simulink model "flexible_joint_v4_rl_Slave_Action_2025"  (R2023b)
settings: Solver=FixedStepAuto  StartTime=0.0  StopTime=40  FixedStep=0.001  RelTol=1e-3
undefined symbols (not defined in the file): DiscIntNeverNeededParam, epsilon, Kmin, LIMIT_SATURATE, NOISE_ADD
libraries: simulink x6, rllib x1
settings Model: Creator=GreenTeam  LastModifiedBy=GreenTeam
settings DataIOCC: InspectSignalLogs=on

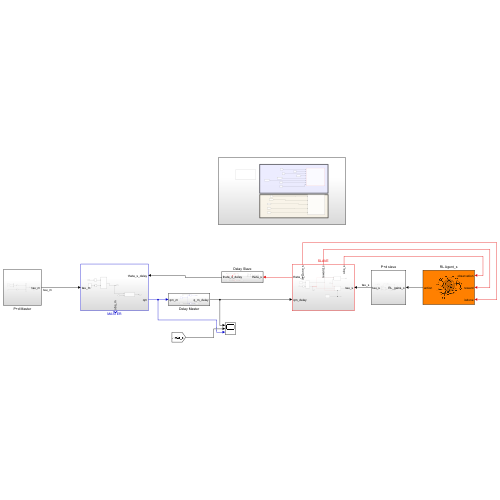
[thumbnail: Simulink's stored preview of the top-level diagram]
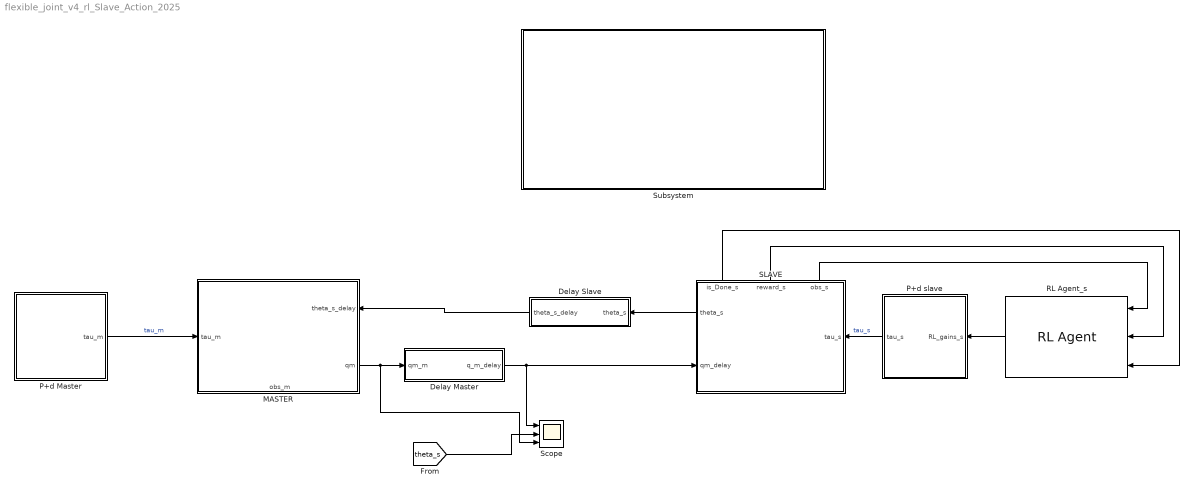
== system flexible_joint_v4_rl_Slave_Action_2025 ==
  Delay Master : Subsystem
  Delay Slave : Subsystem
  MASTER : Subsystem
      settings: PortSchema="{\"entries\":[{\"content\":{\"sides\":[{\"content\":{\"connectorIds\":[\"In1\"]},\"type\":\"ConnectorPlacement.EquallySpacedRectSide\",\"uuid\":\"b129d543-5df5-48a3-934f-a2bf4f7acba4\"},{\"content\":{\"connectorIds\":[\"In2\",\"Out1\"],\"side\":\"RIGHT\"},\"type\":\"ConnectorPlacement.EquallySpacedRectSide\",\"uuid\":\"06efd871-fa3f-497a-8ca9-8980933123ca\"},{\"content\":{\"side\":\"TOP\"},\"type\":\"ConnectorPlacement.EquallySpacedRectSide\",\"uuid\":\"af305e1d-4707-4128-8291-282686c4f98c\"},{\"content\":{\"connectorIds\":[\"Out2\"],\"side\":\"BOTTOM\"},\"type\":\"ConnectorPlacement.EquallySpacedRectSide\",\"uuid\":\"179bfa12-bc3e-4c80-81e3-e51d757695b6\"}]},\"type\":\"ConnectorPlacement.EquallySpacedConnector\",\"uuid\":\"58b08623-3413-4316-b8cd-a4fc96e4577b\"}],\"packageUris\":[\"http://schema.mathworks.com/mf0/Connector/R2020b\"],\"version\":\"1.0\"}"
  P+d Master : Subsystem
  P+d slave : Subsystem
  RL Agent_s : rllib/RL Agent  Agent=agent_s  ExternalActionAsInput=off  ProvideLastAction=off  ProvideCumRwd=off  TreatAsDirectFeedthrough=on  UseStrictObservationDataTypes=off
  SLAVE : Subsystem
      settings: PortSchema="{\"entries\":[{\"content\":{\"sides\":[{\"content\":{\"connectorIds\":[\"In1\"]},\"type\":\"ConnectorPlacement.EquallySpacedRectSide\",\"uuid\":\"b129d543-5df5-48a3-934f-a2bf4f7acba4\"},{\"content\":{\"connectorIds\":[\"Out1\",\"In2\"],\"side\":\"RIGHT\"},\"type\":\"ConnectorPlacement.EquallySpacedRectSide\",\"uuid\":\"06efd871-fa3f-497a-8ca9-8980933123ca\"},{\"content\":{\"connectorIds\":[\"Out2\",\"Out3\",\"Out4\"],\"side\":\"TOP\"},\"type\":\"ConnectorPlacement.EquallySpacedRectSide\",\"uuid\":\"af305e1d-4707-4128-8291-282686c4f98c\"},{\"content\":{\"side\":\"BOTTOM\"},\"type\":\"ConnectorPlacement.EquallySpacedRectSide\",\"uuid\":\"f24c9865-98ea-4837-b1c7-54c0879e04e0\"}]},\"type\":\"ConnectorPlacement.EquallySpacedConnector\",\"uuid\":\"58b08623-3413-4316-b8cd-a4fc96e4577b\"}],\"packageUris\":[\"http://schema.mathworks.com/mf0/Connector/R2020b\"],\"version\":\"1.0\"}"
  Scope : Scope  NumInputPorts=3
  Subsystem : Subsystem
  wires:
  P+d Master/1(tau_m) -> MASTER/1(tau_m)  "tau_m"
  MASTER/1(qm) -> Scope/3, Delay Master/1(qm_m)
  Delay Slave/1(theta_s_delay) -> MASTER/2(theta_s_delay)
  Delay Master/1(q_m_delay) -> Scope/1, SLAVE/2(qm_delay)
  SLAVE/1(theta_s) -> Delay Slave/1(theta_s)
  SLAVE/2(obs_s) -> RL Agent_s/1
  SLAVE/3(reward_s) -> RL Agent_s/2
  SLAVE/4(is_Done_s) -> RL Agent_s/3
  RL Agent_s/1 -> P+d slave/1(RL_gains_s)
  P+d slave/1(tau_s) -> SLAVE/1(tau_s)  "tau_s"
  [theta_s] -> Scope/2

== system flexible_joint_v4_rl_Slave_Action_2025/Delay Master ==
  qm_m : Inport
  Variable Time Delay1 : VariableTransportDelay  MaximumDelay=10  MaximumPoints=499712
  Variable Time Delay5 : VariableTransportDelay  MaximumDelay=10  MaximumPoints=499712
  delay_m : Subsystem
  q_m_delay : Outport
  tag scope: dqm_delay=global
  wires:
  Variable Time Delay5/1 -> q_m_delay/1
  qm_m/1 -> Variable Time Delay5/1
  [dqm] -> Variable Time Delay1/1
  Variable Time Delay1/1 -> [dqm_delay]
  delay_m/1(d) -> Variable Time Delay1/2, Variable Time Delay5/2

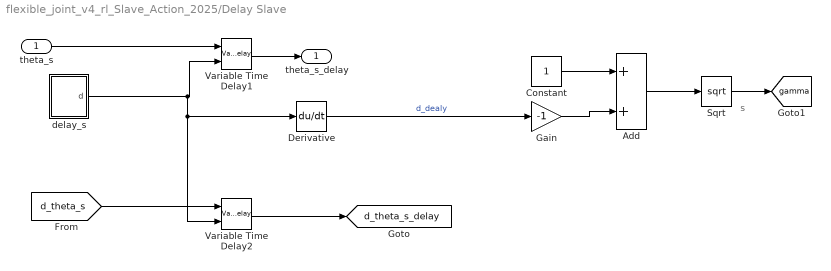
== system flexible_joint_v4_rl_Slave_Action_2025/Delay Slave ==
  note: s
  theta_s : Inport
  Add : Sum
  Constant : Constant
  Derivative : Derivative
  Gain : Gain  Gain=-1
  Sqrt : Sqrt
  Variable Time Delay1 : VariableTransportDelay  MaximumDelay=10  MaximumPoints=499712
  Variable Time Delay2 : VariableTransportDelay  MaximumDelay=10  MaximumPoints=499712
  delay_s : Subsystem
  theta_s_delay : Outport
  tag scope: d_theta_s_delay=global, gamma=global
  wires:
  Variable Time Delay1/1 -> theta_s_delay/1
  theta_s/1 -> Variable Time Delay1/1
  delay_s/1(d) -> Derivative/1, Variable Time Delay2/2, Variable Time Delay1/2
  [d_theta_s] -> Variable Time Delay2/1
  Variable Time Delay2/1 -> [d_theta_s_delay]
  Derivative/1 -> Gain/1  "d_dealy"
  Constant/1 -> Add/1
  Gain/1 -> Add/2
  Add/1 -> Sqrt/1
  Sqrt/1 -> [gamma]

== system flexible_joint_v4_rl_Slave_Action_2025/MASTER ==
  tau_m : Inport
  theta_s_delay : Inport  Port=2
  Master : Subsystem
  Observation : Subsystem
  Saturation1 : Saturate  UpperLimit=LIMIT_SATURATE  LowerLimit=-1*LIMIT_SATURATE
  Saturation2 : Saturate  UpperLimit=LIMIT_SATURATE  LowerLimit=-1*LIMIT_SATURATE
  tauh : Subsystem
  qm : Outport
  obs_m : Outport  Port=2
  wires:
  tauh/1(out) -> Saturation2/1
  tau_m/1 -> Saturation1/1
  Master/1(qm) -> Observation/1(q_m), qm/1
  theta_s_delay/1 -> Observation/2(theta_s_delay)
  Observation/1(observeation) -> obs_m/1
  Saturation2/1 -> Master/2(tau_h)
  Saturation1/1 -> Master/1(tau_m)

== system flexible_joint_v4_rl_Slave_Action_2025/P+d Master ==
  Bm : Gain  Gain=5
  Gain : Gain
  Km : Gain  Gain=5
  Mux2 : Mux  Inputs=2
  Subtract1 : Sum
  tau_m : Outport
  tag scope: tau_m=global
  wires:
  Subtract1/1 -> Gain/1
  Gain/1 -> [tau_m], tau_m/1
  [error_m] -> Km/1
  [dqm_1] -> Mux2/1
  [dqm_2] -> Mux2/2
  Mux2/1 -> Bm/1
  Bm/1 -> Subtract1/1
  Km/1 -> Subtract1/2

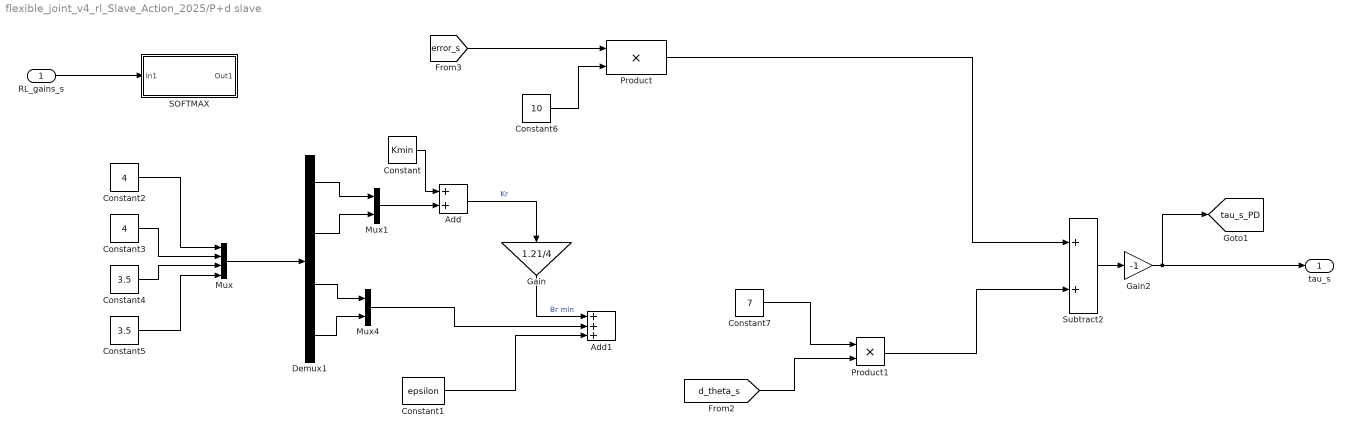
== system flexible_joint_v4_rl_Slave_Action_2025/P+d slave ==
  RL_gains_s : Inport
  Add : Sum
  Add1 : Sum  Inputs=+++
  Constant : Constant  Value=Kmin
  Constant1 : Constant  Value=epsilon
  Constant2 : Constant  Value=4
  Constant3 : Constant  Value=4
  Constant4 : Constant  Value=3.5
  Constant5 : Constant  Value=3.5
  Constant6 : Constant  Value=10
  Constant7 : Constant  Value=7
  Demux1 : Demux
  Gain : Gain  Gain=1.21/4
  Gain2 : Gain  Gain=-1
  Mux : Mux
  Mux1 : Mux  Inputs=2
  Mux4 : Mux  Inputs=2
  Product : Product
  Product1 : Product
  SOFTMAX : Subsystem
  Subtract2 : Sum
  tau_s : Outport
  tag scope: tau_s_PD=global
  wires:
  Subtract2/1 -> Gain2/1
  Gain2/1 -> tau_s/1, [tau_s_PD]
  [error_s] -> Product/1
  Demux1/1 -> Mux1/1
  Demux1/2 -> Mux1/2
  Demux1/3 -> Mux4/1
  Demux1/4 -> Mux4/2
  RL_gains_s/1 -> SOFTMAX/1(In1)
  Mux1/1 -> Add/2
  Constant/1 -> Add/1
  Add/1 -> Gain/1  "Kr"
  Gain/1 -> Add1/1  "Br min"
  Mux4/1 -> Add1/2
  Constant1/1 -> Add1/3
  Product/1 -> Subtract2/1
  Product1/1 -> Subtract2/2
  [d_theta_s] -> Product1/2
  Mux/1 -> Demux1/1
  Constant2/1 -> Mux/1
  Constant5/1 -> Mux/4
  Constant3/1 -> Mux/2
  Constant4/1 -> Mux/3
  Constant6/1 -> Product/2
  Constant7/1 -> Product1/1

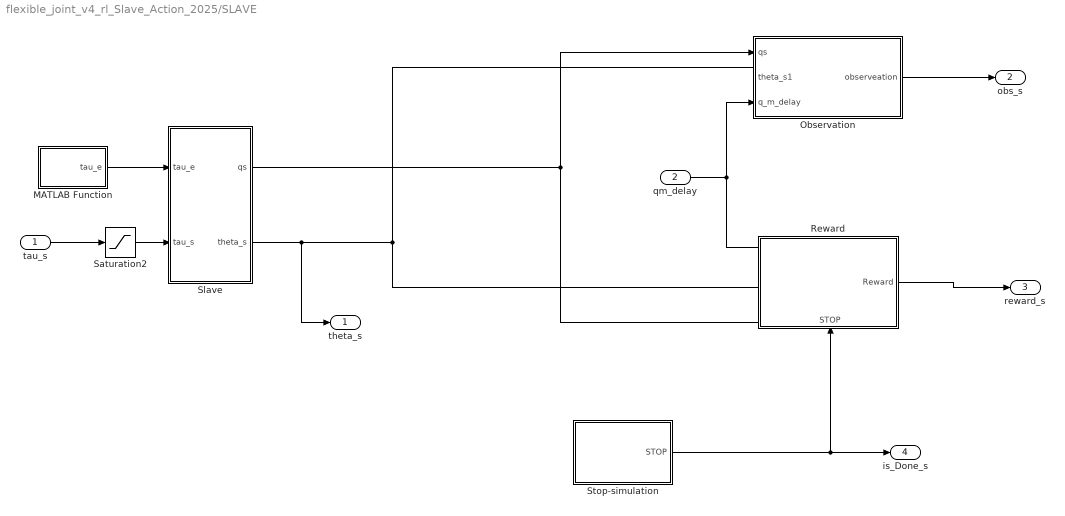
== system flexible_joint_v4_rl_Slave_Action_2025/SLAVE ==
  tau_s : Inport
  qm_delay : Inport  Port=2
  MATLAB Function : MATLAB Function  TreatAsAtomicUnit=on
  Observation : Subsystem
  Reward : Subsystem
      settings: PortSchema="{\"entries\":[{\"content\":{\"sides\":[{\"content\":{},\"type\":\"ConnectorPlacement.EquallySpacedRectSide\",\"uuid\":\"9a737741-b920-4653-b681-b634863af948\"},{\"content\":{\"connectorIds\":[\"Out1\"],\"side\":\"RIGHT\"},\"type\":\"ConnectorPlacement.EquallySpacedRectSide\",\"uuid\":\"0a2b46ef-cff1-47c3-8c56-381f72c27921\"},{\"content\":{\"side\":\"TOP\"},\"type\":\"ConnectorPlacement.EquallySpacedRectSide\",\"uuid\":\"0d3246b3-4748-4708-b0d4-097592cf6e81\"},{\"content\":{\"connectorIds\":[\"In1\"],\"side\":\"BOTTOM\"},\"type\":\"ConnectorPlacement.EquallySpacedRectSide\",\"uuid\":\"566fc9c6-ad4c-440d-8570-c1b5e2d37a92\"}]},\"type\":\"ConnectorPlacement.EquallySpacedConnector\",\"uuid\":\"b2a81796-0154-474c-b467-1f1d418e5717\"}],\"packageUris\":[\"http://schema.mathworks.com/mf0/Connector/R2020b\"],\"version\":\"1.0\"}"
  Saturation2 : Saturate  UpperLimit=LIMIT_SATURATE  LowerLimit=-1*LIMIT_SATURATE
  Slave : Subsystem
  Stop-simulation : Subsystem
  theta_s : Outport
  obs_s : Outport  Port=2
  reward_s : Outport  Port=3
  is_Done_s : Outport  Port=4
  wires:
  MATLAB Function/1(tau_e) -> Slave/1(tau_e)
  tau_s/1 -> Saturation2/1
  Slave/1(qs) -> Observation/1(qs)
  Reward/1(Reward) -> reward_s/1
  Slave/2(theta_s) -> theta_s/1
  qm_delay/1 -> Observation/3(q_m_delay)
  Observation/1(observeation) -> obs_s/1
  Stop-simulation/1(STOP) -> is_Done_s/1, Reward/1(STOP)
  Saturation2/1 -> Slave/2(tau_s)

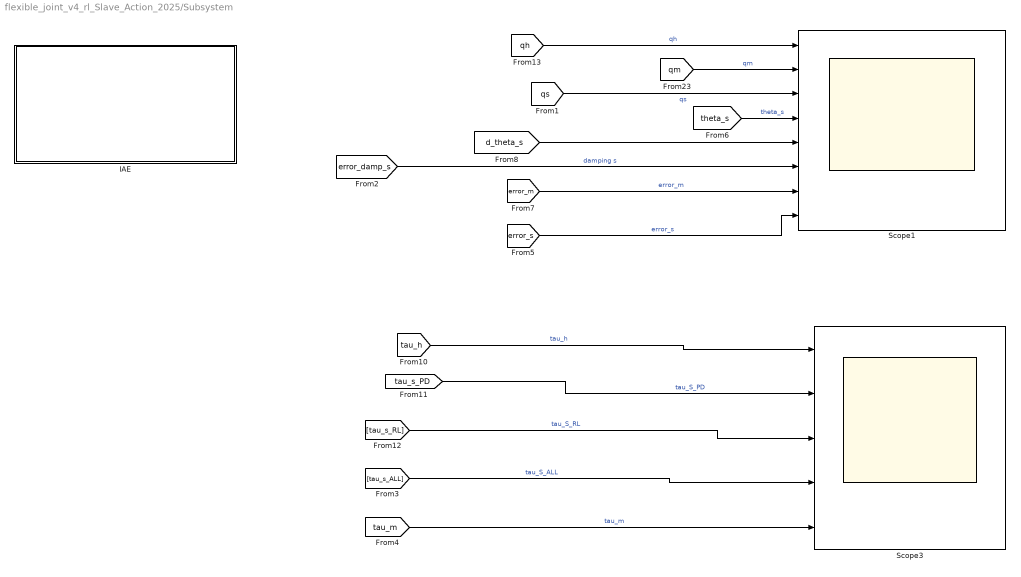
== system flexible_joint_v4_rl_Slave_Action_2025/Subsystem ==
  IAE : Subsystem
  Scope1 : Scope  NumInputPorts=8
  Scope3 : Scope  NumInputPorts=5
  wires:
  [qh] -> Scope1/1  "qh"
  [qm] -> Scope1/2  "qm"
  [error_damp_s] -> Scope1/6  "damping s"
  [error_m] -> Scope1/7  "error_m"
  [error_s] -> Scope1/8  "error_s"
  [qs] -> Scope1/3  "qs"
  [theta_s] -> Scope1/4  "theta_s"
  [d_theta_s] -> Scope1/5
  [tau_s_PD] -> Scope3/2  "tau_S_PD"
  [tau_h] -> Scope3/1  "tau_h"
  [tau_s_RL] -> Scope3/3  "tau_S_RL"
  [tau_s_ALL] -> Scope3/4  "tau_S_ALL"
  [tau_m] -> Scope3/5  "tau_m"

== system flexible_joint_v4_rl_Slave_Action_2025/Delay Master/delay_m ==
  Clock : Clock
  Gain_delay_m : Gain  Gain=0.86907
  MATLAB Function : MATLAB Function  TreatAsAtomicUnit=on
  Scope : Scope
  d : Outport
  wires:
  MATLAB Function/1(y) -> Scope/1, Gain_delay_m/1
  Clock/1 -> MATLAB Function/1(t)
  Gain_delay_m/1 -> d/1

== system flexible_joint_v4_rl_Slave_Action_2025/Delay Slave/delay_s ==
  Clock : Clock
  Gain_delay_s : Gain  Gain=0.73854
  MATLAB Function : MATLAB Function  TreatAsAtomicUnit=on
  d : Outport
  wires:
  Clock/1 -> MATLAB Function/1(t)
  MATLAB Function/1(y) -> Gain_delay_s/1
  Gain_delay_s/1 -> d/1

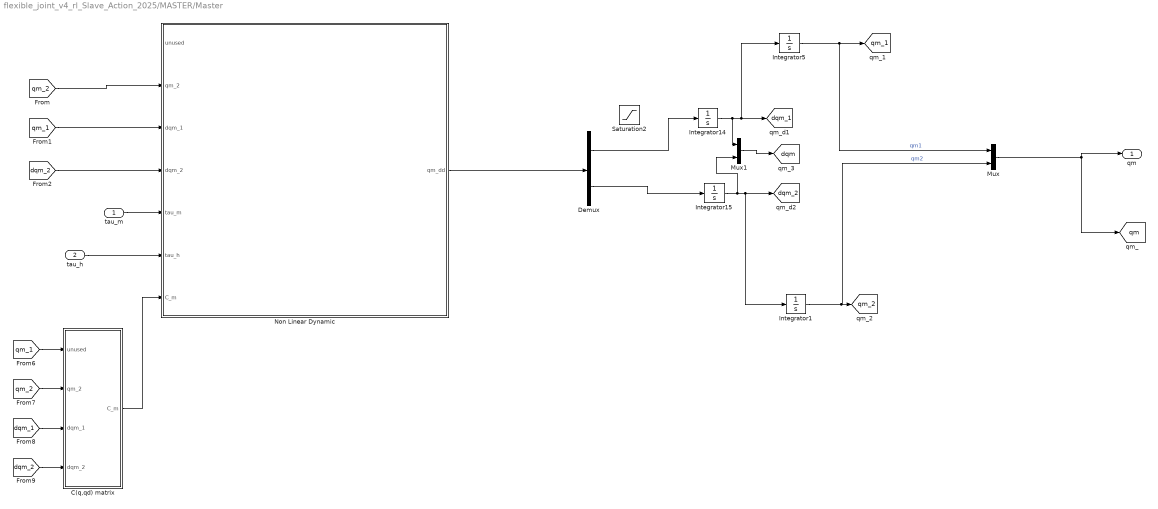
== system flexible_joint_v4_rl_Slave_Action_2025/MASTER/Master ==
  tau_m : Inport
  tau_h : Inport  Port=2
  C(q,qd) matrix : MATLAB Function  TreatAsAtomicUnit=on
  Demux : Demux  Outputs=2
  Integrator1 : Integrator  InitialCondition=1/5
  Integrator14 : Integrator
  Integrator15 : Integrator
  Integrator5 : Integrator  InitialCondition=-1/5
  Mux : Mux  Inputs=2
  Mux1 : Mux  Inputs=2
  Non Linear Dynamic : MATLAB Function  TreatAsAtomicUnit=on
  Saturation2 : Saturate  UpperLimit=1000000  LowerLimit=1000000*-1
  qm : Outport  VectorParamsAs1DForOutWhenUnconnected=off
  tag scope: dqm=global, dqm_1=global, dqm_2=global, qm=global, qm_1=global, qm_2=global
  wires:
  Integrator5/1 -> Mux/1, [qm_1]  "qm1"
  Demux/1 -> Integrator14/1
  Non Linear Dynamic/1(qm_dd) -> Demux/1
  Integrator1/1 -> Mux/2, [qm_2]  "qm2"
  tau_m/1 -> Non Linear Dynamic/5(tau_m)
  Integrator14/1 -> Mux1/1, Integrator5/1, [dqm_1]
  Integrator15/1 -> Mux1/2, Integrator1/1, [dqm_2]
  C(q,qd) matrix/1(C_m) -> Non Linear Dynamic/7(C_m)
  [qm_2] -> Non Linear Dynamic/2(qm_2)
  [dqm_2] -> Non Linear Dynamic/4(dqm_2)
  [qm_1] -> Non Linear Dynamic/3(dqm_1)
  [dqm_1] -> C(q,qd) matrix/3(dqm_1)
  [qm_1] -> C(q,qd) matrix/1(unused)
  [dqm_2] -> C(q,qd) matrix/4(dqm_2)
  [qm_2] -> C(q,qd) matrix/2(qm_2)
  tau_h/1 -> Non Linear Dynamic/6(tau_h)
  Mux1/1 -> [dqm]
  Demux/2 -> Integrator15/1
  Mux/1 -> qm/1, [qm]

== system flexible_joint_v4_rl_Slave_Action_2025/MASTER/Observation ==
  q_m : Inport
  theta_s_delay : Inport  Port=2
  Subtract : Sum  Inputs=+-
  observeation : Outport
  tag scope: error_m=global
  wires:
  q_m/1 -> Subtract/1
  theta_s_delay/1 -> Subtract/2
  Subtract/1 -> [error_m]

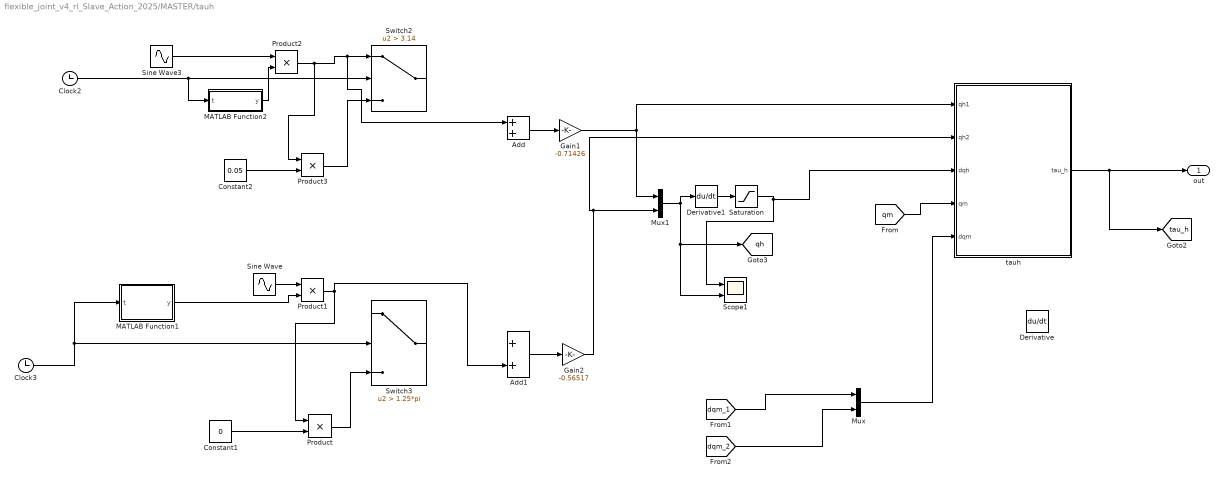
== system flexible_joint_v4_rl_Slave_Action_2025/MASTER/tauh ==
  Add : Sum
  Add1 : Sum
  Clock2 : Clock
  Clock3 : Clock
  Constant1 : Constant  Value=0
  Constant2 : Constant  Value=0.05
  Derivative : Derivative
  Derivative1 : Derivative
  Gain1 : Gain  Gain=-0.71426
  Gain2 : Gain  Gain=-0.56517
  MATLAB Function1 : MATLAB Function  TreatAsAtomicUnit=on
  MATLAB Function2 : MATLAB Function  TreatAsAtomicUnit=on
  Mux : Mux  Inputs=2
  Mux1 : Mux  Inputs=2
  Product{,1..3} (4 alike) : Product
  Saturation : Saturate  UpperLimit=1  LowerLimit=-1
  Scope1 : Scope  NumInputPorts=2
  Sine Wave : Sin  Amplitude=2.5  Frequency=1.6  Phase=0.05  SampleTime=0
  Sine Wave3 : Sin  Amplitude=3  SampleTime=0
  Switch2 : Switch  Criteria=u2 > Threshold  Threshold=3.14  SaturateOnIntegerOverflow=off  InputSameDT=off
  Switch3 : Switch  Criteria=u2 > Threshold  Threshold=1.25*pi  SaturateOnIntegerOverflow=off  InputSameDT=off
  tauh : MATLAB Function  TreatAsAtomicUnit=on
  out : Outport
  tag scope: qh=global, tau_h=global
  wires:
  tauh/1(tau_h) -> [tau_h], out/1
  [dqm_1] -> Mux/1
  [dqm_2] -> Mux/2
  Mux/1 -> tauh/5(dqm)
  [qm] -> tauh/4(qm)
  Mux1/1 -> Scope1/2, [qh], Derivative1/1
  Clock3/1 -> Switch3/2, MATLAB Function1/1(t)
  Clock2/1 -> MATLAB Function2/1(t), Switch2/2
  Add/1 -> Gain1/1
  MATLAB Function1/1(y) -> Product1/2
  Sine Wave/1 -> Product1/1
  Add1/1 -> Gain2/1
  Gain1/1 -> tauh/1(qh1), Mux1/1
  Sine Wave3/1 -> Product2/1
  MATLAB Function2/1(y) -> Product2/2
  Product2/1 -> Product3/1, Add/1, Switch2/1
  Product1/1 -> Product/1, Add1/2
  Derivative1/1 -> Saturation/1
  Saturation/1 -> Scope1/1, tauh/3(dqh)
  Constant1/1 -> Product/2
  Product/1 -> Switch3/3
  Constant2/1 -> Product3/2
  Product3/1 -> Switch2/3
  Gain2/1 -> tauh/2(qh2), Mux1/2

== system flexible_joint_v4_rl_Slave_Action_2025/P+d slave/SOFTMAX ==
  In1 : Inport
  Add : Sum
  Constant : Constant
  Exp : Math
  Log : Math  Operator=log
  Out1 : Outport
  wires:
  Log/1 -> Out1/1
  Constant/1 -> Add/1
  Exp/1 -> Add/2
  In1/1 -> Exp/1
  Add/1 -> Log/1

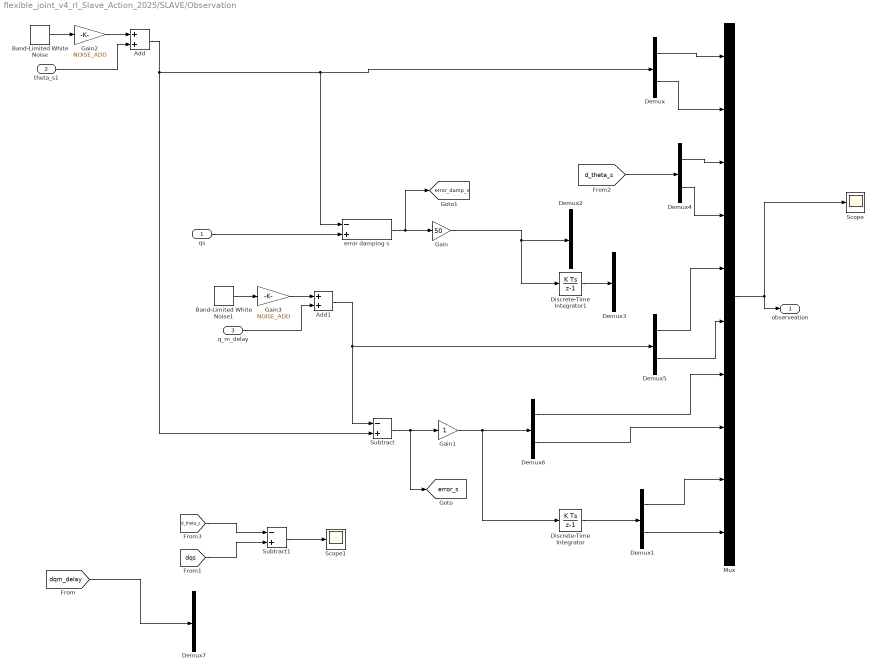
== system flexible_joint_v4_rl_Slave_Action_2025/SLAVE/Observation ==
  qs : Inport
  theta_s1 : Inport  Port=2
  q_m_delay : Inport  Port=3
  Add : Sum
  Add1 : Sum
  Band-Limited White Noise : simulink/Sources/Band-Limited White Noise  Cov=[0.005]  Ts=0.01  seed=[23341]
  Band-Limited White Noise1 : simulink/Sources/Band-Limited White Noise  Cov=[0.005]  Ts=0.01  seed=[23341]
  Demux{,1..7} (8 alike) : Demux  Outputs=2
  Discrete-Time Integrator : DiscreteIntegrator  SampleTime=-1  ICPrevOutput=DiscIntNeverNeededParam  ICPrevScaledInput=DiscIntNeverNeededParam
  Discrete-Time Integrator1 : DiscreteIntegrator  SampleTime=-1  ICPrevOutput=DiscIntNeverNeededParam  ICPrevScaledInput=DiscIntNeverNeededParam
  Gain : Gain  Gain=50
  Gain1 : Gain
  Gain2 : Gain  Gain=NOISE_ADD
  Gain3 : Gain  Gain=NOISE_ADD
  Mux : Mux  Inputs=10
  Scope : Scope
  Scope1 : Scope
  Subtract : Sum  Inputs=-+
  Subtract1 : Sum  Inputs=-+
  error damping s : Sum  Inputs=-+
  observeation : Outport
  tag scope: error_damp_s=global, error_s=global
  wires:
  Discrete-Time Integrator/1 -> Demux1/1
  Mux/1 -> Scope/1, observeation/1
  Add/1 -> Subtract/2, error damping s/1, Demux/1
  [d_theta_s] -> Demux4/1
  qs/1 -> error damping s/2
  Discrete-Time Integrator1/1 -> Demux3/1
  error damping s/1 -> [error_damp_s], Gain/1
  [dqm_delay] -> Demux7/1
  Subtract/1 -> [error_s], Gain1/1
  Gain/1 -> Discrete-Time Integrator1/1, Demux2/1
  Demux/1 -> Mux/1
  Demux/2 -> Mux/2
  Demux4/1 -> Mux/3
  Demux4/2 -> Mux/4
  Demux5/1 -> Mux/5
  Demux5/2 -> Mux/6
  Gain1/1 -> Discrete-Time Integrator/1, Demux6/1
  [dqs] -> Subtract1/2
  [d_theta_s] -> Subtract1/1
  Subtract1/1 -> Scope1/1
  Demux6/1 -> Mux/7
  Demux6/2 -> Mux/8
  Demux1/1 -> Mux/9
  Demux1/2 -> Mux/10
  Band-Limited White Noise/1 -> Gain2/1
  Gain2/1 -> Add/1
  theta_s1/1 -> Add/2
  Band-Limited White Noise1/1 -> Gain3/1
  q_m_delay/1 -> Add1/2
  Gain3/1 -> Add1/1
  Add1/1 -> Subtract/1, Demux5/1

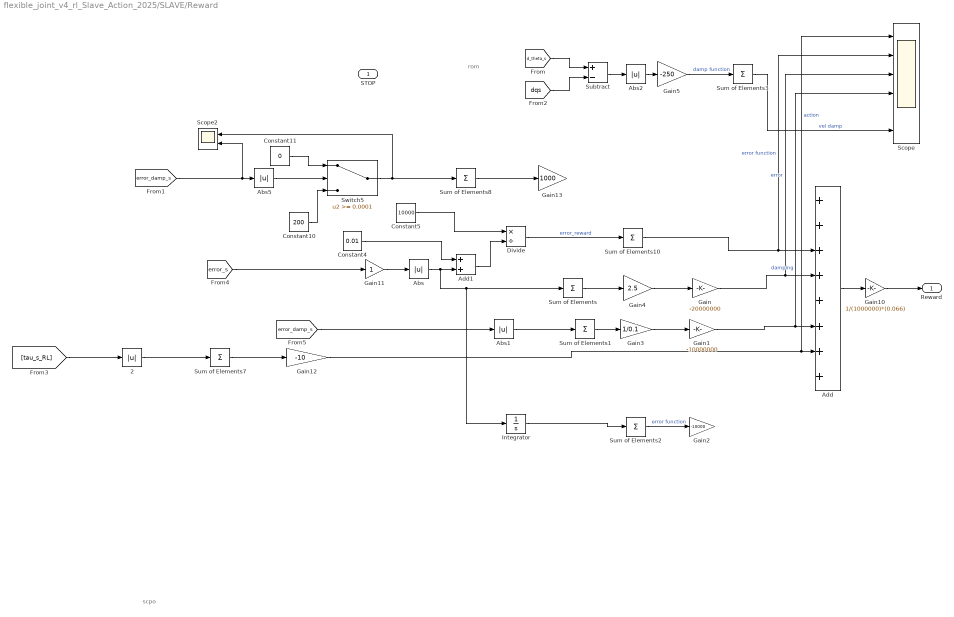
== system flexible_joint_v4_rl_Slave_Action_2025/SLAVE/Reward ==
  note: rom
  note: scpo
  STOP : Inport
  " 2" : Abs  SaturateOnIntegerOverflow=off
  Abs{,1..2,5} (4 alike) : Abs  SaturateOnIntegerOverflow=off
  Add : Sum  Inputs=++++++++
  Add1 : Sum
  Constant10 : Constant  Value=200
  Constant11 : Constant  Value=0
  Constant4 : Constant  Value=0.01
  Constant5 : Constant  Value=10000
  Divide : Product  Inputs=*/
  Gain : Gain  Gain=-20000000
  Gain1 : Gain  Gain=-10000000
  Gain10 : Gain  Gain=1/(1000000)*(0.066)
  Gain11 : Gain
  Gain12 : Gain  Gain=-10
  Gain13 : Gain  Gain=1000
  Gain2 : Gain  Gain=-10000
  Gain3 : Gain  Gain=1/0.1
  Gain4 : Gain  Gain=2.5
  Gain5 : Gain  Gain=-250
  Integrator : Integrator
  Scope : Scope  NumInputPorts=6
  Scope2 : Scope  NumInputPorts=2
  Subtract : Sum  Inputs=+-
  Sum of Elements{,1..3,7..8,10} (7 alike) : Sum  Inputs=+
  Switch5 : Switch  Threshold=0.0001  SaturateOnIntegerOverflow=off  InputSameDT=off
  Reward : Outport
  wires:
  Sum of Elements/1 -> Gain4/1
  Gain4/1 -> Gain/1
  Sum of Elements1/1 -> Gain3/1
  Gain3/1 -> Gain1/1
  Abs1/1 -> Sum of Elements1/1
  [error_damp_s] -> Abs1/1
  Add/1 -> Gain10/1
  Gain10/1 -> Reward/1
  Abs/1 -> Integrator/1, Sum of Elements/1, Add1/2
  Constant4/1 -> Add1/1
  Add1/1 -> Divide/2
  Constant5/1 -> Divide/1
  Gain11/1 -> Abs/1
  [error_s] -> Gain11/1
  [tau_s_RL] -> " 2"/1
  Sum of Elements7/1 -> Gain12/1
  Gain12/1 -> Scope/1, Add/7  "action"
  [error_damp_s] -> Abs5/1, Scope2/2
  Constant10/1 -> Switch5/3
  Constant11/1 -> Switch5/1
  Switch5/1 -> Sum of Elements8/1, Scope2/1
  Sum of Elements8/1 -> Gain13/1
  Divide/1 -> Sum of Elements10/1  "error_reward"
  Abs5/1 -> Switch5/2
  " 2"/1 -> Sum of Elements7/1
  Gain1/1 -> Scope/4, Add/6  "damping"
  Sum of Elements10/1 -> Scope/2, Add/3  "error function"
  Gain/1 -> Scope/3, Add/4  "error"
  Integrator/1 -> Sum of Elements2/1
  Sum of Elements2/1 -> Gain2/1  "error function"
  [d_theta_s] -> Subtract/1
  [dqs] -> Subtract/2
  Subtract/1 -> Abs2/1
  Sum of Elements3/1 -> Scope/6  "vel damp"
  Abs2/1 -> Gain5/1
  Gain5/1 -> Sum of Elements3/1  "damp function"

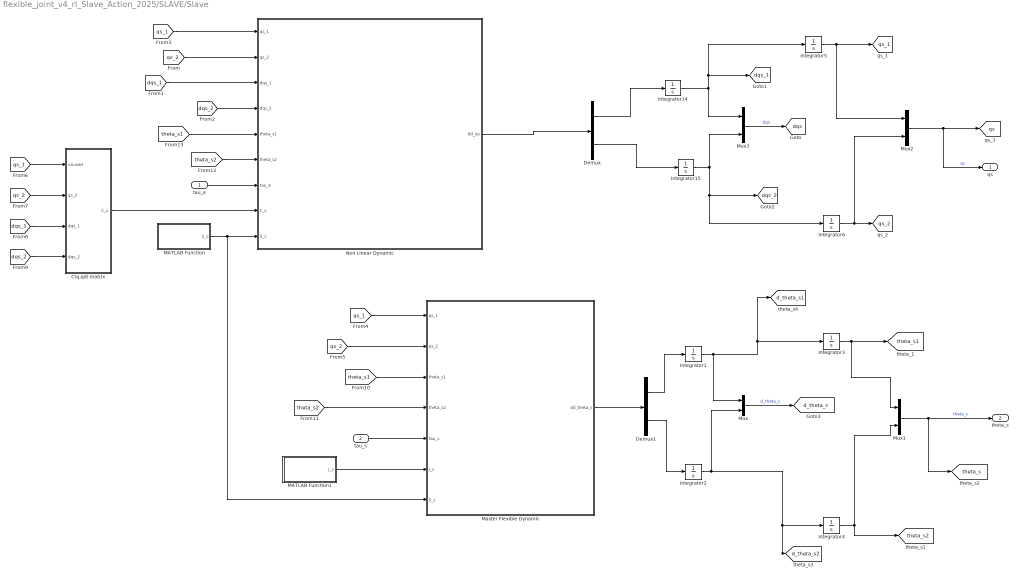
== system flexible_joint_v4_rl_Slave_Action_2025/SLAVE/Slave ==
  tau_e : Inport
  tau_s : Inport  Port=2
  C(q,qd) matrix : MATLAB Function  TreatAsAtomicUnit=on
  Demux : Demux  Outputs=2
  Demux1 : Demux  Outputs=2
  Integrator{1..4,14..15} (6 alike) : Integrator
  Integrator5 : Integrator  InitialCondition=-0.1
  Integrator6 : Integrator  InitialCondition=0.1
  MATLAB Function : MATLAB Function  TreatAsAtomicUnit=on
  MATLAB Function1 : MATLAB Function  TreatAsAtomicUnit=on
  Master Flexible Dynamic : MATLAB Function  TreatAsAtomicUnit=on
  Mux{,1..3} (4 alike) : Mux  Inputs=2
  Non Linear Dynamic : MATLAB Function  TreatAsAtomicUnit=on
  qs : Outport
  theta_s : Outport  Port=2
  tag scope: d_theta_s1=global, d_theta_s2=global, d_theta_s=global, dqs=global, dqs_1=global, dqs_2=global, qs=global, qs_1=global, qs_2=global, theta_s1=global, theta_s2=global, theta_s=global
  wires:
  [qs_2] -> C(q,qd) matrix/2(qs_2)
  [dqs_2] -> C(q,qd) matrix/4(dqs_2)
  [qs_1] -> C(q,qd) matrix/1(unused)
  [dqs_1] -> C(q,qd) matrix/3(dqs_1)
  [dqs_1] -> Non Linear Dynamic/3(dqs_1)
  [dqs_2] -> Non Linear Dynamic/4(dqs_2)
  [qs_2] -> Non Linear Dynamic/2(qs_2)
  Demux/2 -> Integrator15/1
  Integrator15/1 -> Mux3/2, [dqs_2], Integrator6/1
  Integrator6/1 -> Mux2/2, [qs_2]
  Non Linear Dynamic/1(dd_qs) -> Demux/1
  Demux/1 -> Integrator14/1
  Mux2/1 -> [qs], qs/1  "qs"
  Integrator5/1 -> Mux2/1, [qs_1]
  C(q,qd) matrix/1(C_s) -> Non Linear Dynamic/8(C_s)
  MATLAB Function/1(S_s) -> Non Linear Dynamic/9(S_s), Master Flexible Dynamic/7(S_s)
  [qs_1] -> Non Linear Dynamic/1(qs_1)
  MATLAB Function1/1(J_s) -> Master Flexible Dynamic/6(J_s)
  Integrator3/1 -> Mux1/1, [theta_s1]
  Integrator1/1 -> Mux/1, Integrator3/1, [d_theta_s1]
  Demux1/1 -> Integrator1/1
  Master Flexible Dynamic/1(dd_theta_s) -> Demux1/1
  Integrator4/1 -> [theta_s2], Mux1/2
  Integrator2/1 -> Mux/2, [d_theta_s2], Integrator4/1
  Mux1/1 -> [theta_s], theta_s/1  "theta_s"
  Demux1/2 -> Integrator2/1
  [qs_1] -> Master Flexible Dynamic/1(qs_1)
  [qs_2] -> Master Flexible Dynamic/2(qs_2)
  [theta_s1] -> Master Flexible Dynamic/3(theta_s1)
  [theta_s2] -> Master Flexible Dynamic/4(theta_s2)
  [theta_s2] -> Non Linear Dynamic/6(theta_s2)
  [theta_s1] -> Non Linear Dynamic/5(theta_s1)
  tau_e/1 -> Non Linear Dynamic/7(tau_e)
  tau_s/1 -> Master Flexible Dynamic/5(tau_s)
  Integrator14/1 -> Mux3/1, [dqs_1], Integrator5/1
  Mux3/1 -> [dqs]  "dqs"
  Mux/1 -> [d_theta_s]  "d_theta_s"

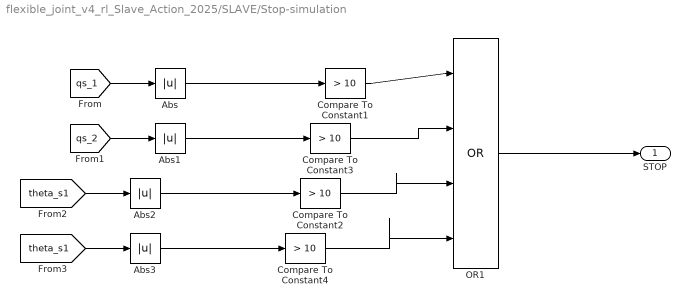
== system flexible_joint_v4_rl_Slave_Action_2025/SLAVE/Stop-simulation ==
  Abs{,1..3} (4 alike) : Abs  SaturateOnIntegerOverflow=off
  Compare To Constant{1..4} (4 alike) : simulink/Logic and Bit Operations/Compare To Constant  relop=>  const=10  OutDataTypeStr=boolean
  OR1 : Logic  Operator=OR  Inputs=4  IconShape=distinctive  AllPortsSameDT=off  OutDataTypeStr=boolean
  STOP : Outport  VectorParamsAs1DForOutWhenUnconnected=off
  wires:
  OR1/1 -> STOP/1
  [qs_1] -> Abs/1
  [qs_2] -> Abs1/1
  Abs/1 -> Compare To Constant1/1
  Abs1/1 -> Compare To Constant3/1
  Compare To Constant1/1 -> OR1/1
  Compare To Constant3/1 -> OR1/2
  Abs3/1 -> Compare To Constant4/1
  Abs2/1 -> Compare To Constant2/1
  [theta_s1] -> Abs3/1
  [theta_s1] -> Abs2/1
  Compare To Constant2/1 -> OR1/3
  Compare To Constant4/1 -> OR1/4

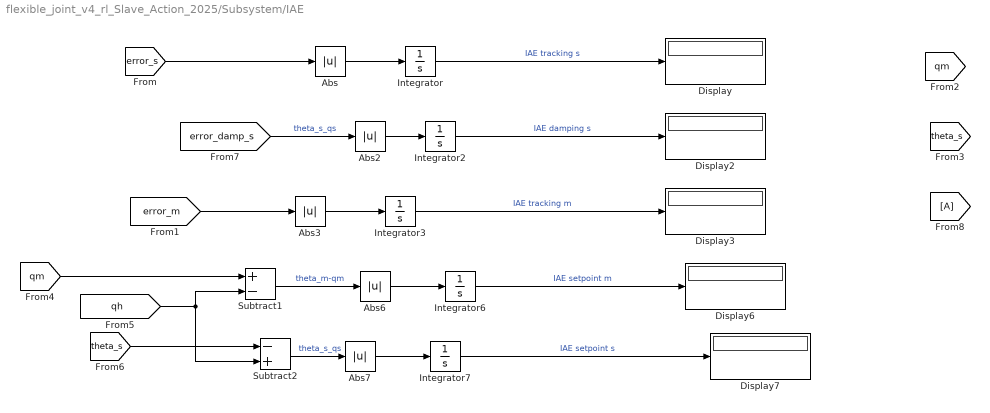
== system flexible_joint_v4_rl_Slave_Action_2025/Subsystem/IAE ==
  Abs{,2..3,6..7} (5 alike) : Abs  SaturateOnIntegerOverflow=off
  Display{,2..3,6..7} (5 alike) : Display
  From8 : From
  Integrator{,2..3,6..7} (5 alike) : Integrator
  Subtract1 : Sum  Inputs=+-
  Subtract2 : Sum  Inputs=-+
  wires:
  Integrator2/1 -> Display2/1  "IAE damping s"
  Abs/1 -> Integrator/1
  [error_damp_s] -> Abs2/1  "theta_s_qs"
  Integrator/1 -> Display/1  "IAE tracking s"
  Abs2/1 -> Integrator2/1
  [error_s] -> Abs/1
  [error_m] -> Abs3/1
  Integrator3/1 -> Display3/1  "IAE tracking m"
  Abs3/1 -> Integrator3/1
  [qm] -> Subtract1/1
  Abs7/1 -> Integrator7/1
  [qh] -> Subtract2/2, Subtract1/2
  Integrator6/1 -> Display6/1  "IAE setpoint m"
  Subtract1/1 -> Abs6/1  "theta_m-qm"
  [theta_s] -> Subtract2/1
  Abs6/1 -> Integrator6/1
  Subtract2/1 -> Abs7/1  "theta_s_qs"
  Integrator7/1 -> Display7/1  "IAE setpoint s"

== matlab function flexible_joint_v4_rl_Slave_Action_2025/MASTER/tauh/MATLAB Function1 ==
  data: t input; y output
function y = exp_decay(t)
alpha=0.04;
y = exp(-alpha*t);

== matlab function flexible_joint_v4_rl_Slave_Action_2025/MASTER/tauh/tauh ==
  data: qh1 input; qh2 input; dqh input; qm input; tau_h output; dqm input
function tau_h = spring_damper(qh1,qh2,dqh,qm,dqm)

Kh=1000;
Dh=2;

qh=[qh1;qh2];
%dqh=[dqh1;dqh2];
tau_h=Kh*(qh-qm)-Dh*(dqh-dqm);


end

== matlab function flexible_joint_v4_rl_Slave_Action_2025/MASTER/Master/Non Linear Dynamic ==
  data: unused input; qm_2 input; dqm_1 input; dqm_2 input; tau_m input; tau_h input; qm_dd output; C_m input
function qm_dd =fcn(~,qm_2,dqm_1,dqm_2,tau_m,tau_h,C_m)

% Phyiscal Parameters
Lm1 = 0.38;                                          %Master_first_link_length
Lm2 = 0.38;                                          %Master_second_link_length
mm1 = 0.5;                                           %Master_first_link_mass
mm2 = 0.35;                                           %Master_second_link_mass


dqm=[dqm_1;dqm_2];
alpha_m=(Lm2^2)*mm2+(Lm1^2)*(mm1+mm2);
betha_m=Lm1*Lm2*mm2;
delta_m=(Lm2^2)*mm2;

M_m_11= alpha_m + 2*betha_m*cos(qm_2);  
M_m_12= delta_m + betha_m * cos(qm_2);
M_m_21= M_m_12;
M_m_22= delta_m;
M_m = [M_m_11 M_m_12; M_m_21 M_m_22];
qm_dd = inv(M_m)*( -tau_m -(C_m * dqm ) + tau_h );
end

== matlab function flexible_joint_v4_rl_Slave_Action_2025/Delay Master/delay_m/MATLAB Function ==
  data: t input; y output
function y = reconstructed_signal(t)
    % Given data
    DC_offset = 0.9613462407597305;
    sine_amplitudes = [-0.02000659, -0.02349457, 0.00067474, 0.00159032, 0.00129016, -0.00135477, -0.00022001, 0.00097632, 0.00021585, 0.00014519, -0.00020833, -0.00056968, -0.00031181, 0.00016964, 0.0003376, -0.00022124];
    cosine_amplitudes = [-0.02556397, 0.00393168, -0.0052079, 0.00220769, 0.00300956, 0.00160663, -0.00018929, -0.00031848, -0.00019025, -0.00022222, -0.00010147, 0.00019351, -0.00030343, 0.0001225, 0.00015061, 0.00039704];
    frequencies = [0.24299065416927243, 0.48598130833854486, 0.7289719625078173, 0.9719626166770897, 1.2149532708463622, 1.4579439250156345, 1.7009345791849069, 1.9439252333541794, 2.186915887523452, 2.4299065416927244, 2.6728971958619967, 2.915887850031269, 3.1588785042005414, 3.4018691583698137, 3.6448598125390865, 3.887850466708359];
    
    % Number of terms
    N = length(sine_amplitudes);
    
    % Initialize the signal
    y = DC_offset * ones(size(t));
    
    % Add sine and cosine terms
    for k = 1:N
        y = y + sine_amplitudes(k) * sin(2 * pi * frequencies(k) * t) + cosine_amplitudes(k) * cos(2 * pi * frequencies(k) * t);
    end
    
end

== matlab function flexible_joint_v4_rl_Slave_Action_2025/SLAVE/Slave/C(q,qd) matrix ==
  data: unused input; qs_2 input; dqs_1 input; C_s output; dqs_2 input
function C_s = fcn(~,qs_2,dqs_1,dqs_2)

% Phyiscal Parameters
Ls1 = 0.38;                                          %Slave_first_link_length
Ls2 = 0.38;                                          %Slave_second_link_length
ms1 = 0.5;                                           %Slave_first_link_mass
ms2 = 0.35;                                          %Slave_second_link_mass

betha_s=Ls1*Ls2*ms2;

C_s_11 = -1*betha_s*sin(qs_2)*dqs_2;
C_s_12 = -1*betha_s*sin(qs_2)*(dqs_1+dqs_2);
C_s_21 =  betha_s*sin(qs_2)*dqs_1;
C_s_22 =  0;
C_s= [C_s_11 C_s_12; C_s_21 C_s_22];
end

== matlab function flexible_joint_v4_rl_Slave_Action_2025/SLAVE/Slave/MATLAB Function ==
  data: S_s output
function S_s = Stifness_Matrix()
    % This function creates a 2x2 identity matrix scaled by 500

    % Create a 2x2 identity matrix
    I = eye(2);
    
    % Scale the identity matrix by 500
    S_s = 100 * I;
end

== matlab function flexible_joint_v4_rl_Slave_Action_2025/SLAVE/Slave/Master Flexible Dynamic ==
  data: qs_1 input; qs_2 input; theta_s1 input; dd_theta_s output; theta_s2 input; tau_s input; J_s input; S_s input
function dd_theta_s = Flex_Body_Slave(qs_1,qs_2,theta_s1,theta_s2,tau_s,J_s,S_s)

qs=[qs_1;qs_2];
theta_s=[theta_s1;theta_s2];


dd_theta_s = inv(J_s)*(tau_s - S_s*(theta_s-qs));

end

== matlab function flexible_joint_v4_rl_Slave_Action_2025/SLAVE/Slave/MATLAB Function1 ==
  data: J_s output
function J_s = Inertia_Matrix()

    % Create a 2x2 identity matrix
    I = eye(2);
    % Scale the identity matrix by 500
    J_s = 0.3 * I;
end

== matlab function flexible_joint_v4_rl_Slave_Action_2025/SLAVE/MATLAB Function ==
  data: tau_e output
function tau_e = fcn()

tau_e=[0;0];

== matlab function flexible_joint_v4_rl_Slave_Action_2025/SLAVE/Slave/Non Linear Dynamic ==
  data: qs_1 input; qs_2 input; dqs_1 input; dqs_2 input; theta_s1 input; theta_s2 input; dd_qs output; tau_e input; C_s input; S_s input
function dd_qs =Rigid_Body_Slave(qs_1,qs_2,dqs_1,dqs_2,theta_s1,theta_s2,tau_e,C_s,S_s)

% Phyiscal Parameters
Ls1 = 0.38;                                          %Slave_first_link_length
Ls2 = 0.38;                                          %Slave_second_link_length
ms1 = 0.5;                                           %Slave_first_link_mass
ms2 = 0.35;                                          %Slave_second_link_mass

qs=[qs_1;qs_2];
theta_s=[theta_s1;theta_s2];
dqs=[dqs_1;dqs_2];
alpha_s=(Ls2^2)*ms2+(Ls1^2)*(ms1+ms2);
betha_s=Ls1*Ls2*ms2;
delta_s=(Ls2^2)*ms2;

M_s_11= alpha_s + 2*betha_s*cos(qs_2);  
M_s_12= delta_s + betha_s * cos(qs_2);
M_s_21= M_s_12;
M_s_22= delta_s;
M_s = [M_s_11 M_s_12; M_s_21 M_s_22];
dd_qs= inv(M_s)*(- tau_e  - (C_s * dqs ) - (S_s*(qs-theta_s)));
end

== matlab function flexible_joint_v4_rl_Slave_Action_2025/Delay Slave/delay_s/MATLAB Function ==
  data: t input; y output
function y = reconstructed_signal(t)
    % Given data
    DC_offset = 0.9613462407597305;
    sine_amplitudes = [-0.02000659, -0.02349457, 0.00067474, 0.00159032, 0.00129016, -0.00135477, -0.00022001, 0.00097632, 0.00021585, 0.00014519, -0.00020833, -0.00056968, -0.00031181, 0.00016964, 0.0003376, -0.00022124];
    cosine_amplitudes = [-0.02556397, 0.00393168, -0.0052079, 0.00220769, 0.00300956, 0.00160663, -0.00018929, -0.00031848, -0.00019025, -0.00022222, -0.00010147, 0.00019351, -0.00030343, 0.0001225, 0.00015061, 0.00039704];
    frequencies = [0.24299065416927243, 0.48598130833854486, 0.7289719625078173, 0.9719626166770897, 1.2149532708463622, 1.4579439250156345, 1.7009345791849069, 1.9439252333541794, 2.186915887523452, 2.4299065416927244, 2.6728971958619967, 2.915887850031269, 3.1588785042005414, 3.4018691583698137, 3.6448598125390865, 3.887850466708359];
    
    % Number of terms
    N = length(sine_amplitudes);
    
    % Initialize the signal
    y = DC_offset * ones(size(t));
    
    % Add sine and cosine terms
    for k = 1:N
        y = y + sine_amplitudes(k) * sin(2 * pi * frequencies(k) * t) + cosine_amplitudes(k) * cos(2 * pi * frequencies(k) * t);
    end
    
end

== matlab function flexible_joint_v4_rl_Slave_Action_2025/MASTER/Master/C(q,qd) matrix ==
  data: unused input; qm_2 input; dqm_1 input; C_m output; dqm_2 input
function C_m = fcn(~,qm_2,dqm_1,dqm_2)

% Phyiscal Parameters
Lm1 = 0.38;                                          %Master_first_link_length
Lm2 = 0.38;                                          %Master_second_link_length
mm1 = 3.947368;                                           %Master_first_link_mass
mm2 = 0.62326;                                           %Master_second_link_mass

betha_m=Lm1*Lm2*mm2;

C_m_11 = -1*betha_m*sin(qm_2)*dqm_2;
C_m_12 = -betha_m*sin(qm_2)*(dqm_1+dqm_2);
C_m_21 =  betha_m*sin(qm_2)*dqm_1;
C_m_22 =  0;
C_m = [C_m_11 C_m_12; C_m_21 C_m_22];
end

== matlab function flexible_joint_v4_rl_Slave_Action_2025/MASTER/tauh/MATLAB Function2 ==
  data: t input; y output
function y = exp_decay(t)
alpha=0.05;
y = exp(-alpha*t);
